simulink model "pset1_simulink"  (R2022a)
settings: Solver=VariableStepAuto  StartTime=0.0  StopTime=10.0  RelTol=1e-3
values from neighbouring files (symbols this model uses):
  a = inf    [inert2OE.m]    (also in pset1.m = state(1); pset2.m = 1 / (2 / norm(pos) - norm(vel)^2 / mu))
  e = norm(e_vec)    [inert2OE.m]    (also in pset1.m = sqrt(1 - p / a); pset2.m = sqrt(1 - p / a); pset4.m = sqrt(oe_c_mean_pert(i, 3)^2 + oe_c_mean_pert(i, 4)^2))
  i = acos(h_vec(3)/h)    [inert2OE.m]    (also in pset1.m = state(4); pset2.m = atan2(sqrt(W(1)^2 + W(2)^2), W(3)); pset5_NR.m = 1)
  mu = 3.986004418e5    (= 398600.4418)    [pset1.m]    (also in pset2.m = 398600.435436; pset3.m = 398600.435436; pset3_problem1.m = 398600.435436; pset3_problem2.m = 398600.435436)
  omega = 2*pi - omega    [inert2OE.m]    (also in pset1.m = u - nu; pset2.m = wrapTo2Pi(u - nu); pset4.m = atan2(oe_c_mean_pert(i,4), oe_c_mean_pert(i, 3)))
  RAAN = atan2(W(1), - W(2))    [pset1.m]    (also in pset2.m)
  true_anom = 0    [pset1.m]
settings Model: Creator=pauli  LastModifiedBy=pauli

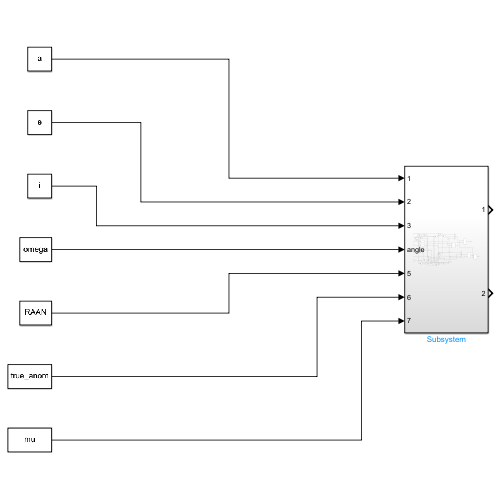
[thumbnail: Simulink's stored preview of the top-level diagram]
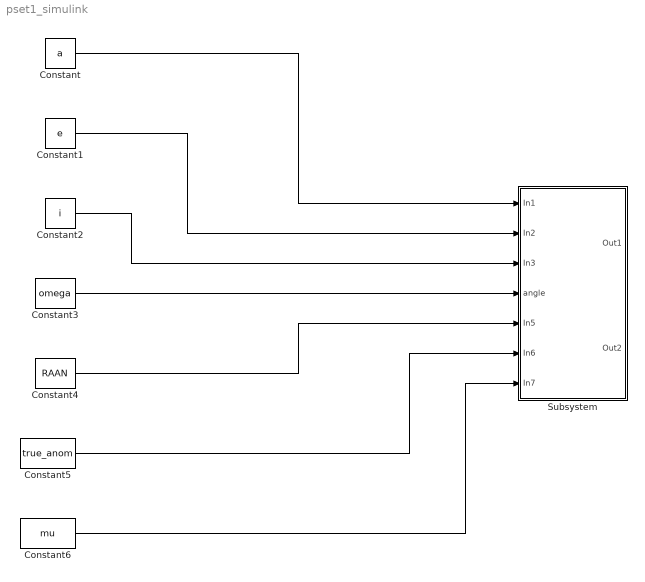
== system pset1_simulink ==
  Constant : Constant  Value=a
  Constant1 : Constant  Value=e
  Constant2 : Constant  Value=i
  Constant3 : Constant  Value=omega
  Constant4 : Constant  Value=RAAN
  Constant5 : Constant  Value=true_anom
  Constant6 : Constant  Value=mu
  Subsystem : Subsystem
  wires:
  Constant/1 -> Subsystem/1(In1)
  Constant1/1 -> Subsystem/2(In2)
  Constant2/1 -> Subsystem/3(In3)
  Constant3/1 -> Subsystem/4(angle)
  Constant4/1 -> Subsystem/5(In5)
  Constant5/1 -> Subsystem/6(In6)
  Constant6/1 -> Subsystem/7(In7)

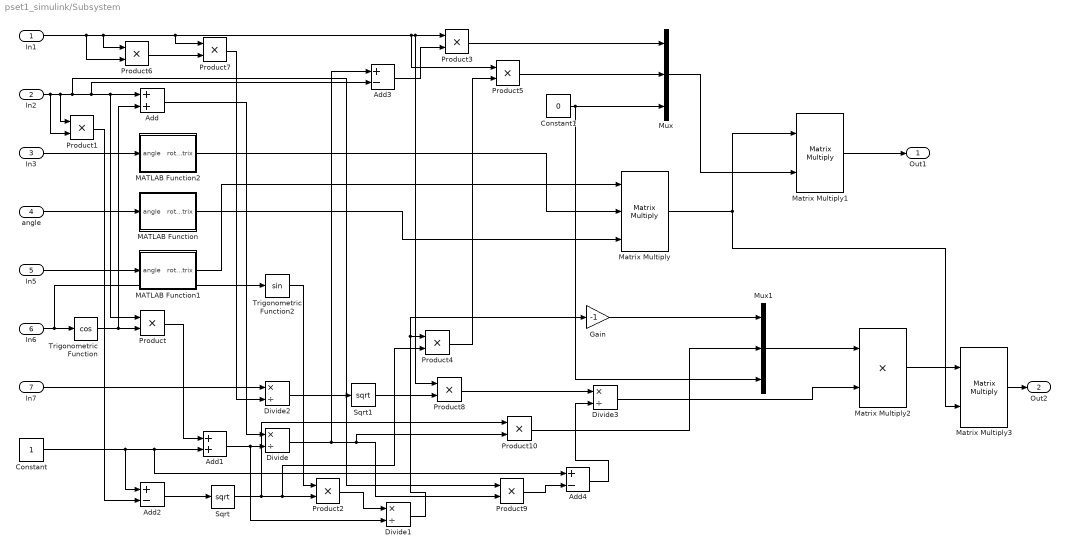
== system pset1_simulink/Subsystem ==
  In1 : Inport  Unit=km
      settings: VarSizeSig=Yes
  In2 : Inport  Port=2
  In3 : Inport  Port=3
  angle : Inport  Port=4
  In5 : Inport  Port=5
  In6 : Inport  Port=6
  In7 : Inport  Port=7
  Add : Sum
  Add1 : Sum
  Add2 : Sum  Inputs=+-
  Add3 : Sum  Inputs=+-
  Add4 : Sum  Inputs=+-
  Constant : Constant
  Constant1 : Constant  Value=0
  Divide{,1..3} (4 alike) : Product  Inputs=*/
  Gain : Gain  Gain=-1
  MATLAB Function : MATLAB Function  TreatAsAtomicUnit=on
  MATLAB Function1 : MATLAB Function  TreatAsAtomicUnit=on
  MATLAB Function2 : MATLAB Function  TreatAsAtomicUnit=on
  Matrix Multiply : Product  Inputs=3  Multiplication=Matrix(*)
  Matrix Multiply1 : Product  Multiplication=Matrix(*)
  Matrix Multiply2 : Product
  Matrix Multiply3 : Product  Multiplication=Matrix(*)
  Mux : Mux  Inputs=3
  Mux1 : Mux  Inputs=3
  Product{,1..10} (11 alike) : Product
  Sqrt : Sqrt
  Sqrt1 : Sqrt
  Trigonometric Function : Trigonometry  Operator=cos
  Trigonometric Function2 : Trigonometry
  Out1 : Outport
  Out2 : Outport  Port=2
  wires:
  In6/1 -> Trigonometric Function2/1, Trigonometric Function/1
  In2/1 -> Product1/2, Product1/1, Product9/1, Add3/2, Product/1, Add/1
  Trigonometric Function/1 -> Product/2, Add/2
  Constant/1 -> Add2/1, Add4/1, Add1/2
  Product/1 -> Add1/1
  Add1/1 -> Divide1/2, Divide/2
  Add/1 -> Divide/1
  Divide/1 -> Add3/1, Product10/2, Product9/2
  Product1/1 -> Add2/2
  Add2/1 -> Sqrt/1
  Sqrt/1 -> Product10/1, Product4/2, Product2/2
  Trigonometric Function2/1 -> Product2/1
  Product2/1 -> Divide1/1
  Divide1/1 -> Gain/1, Product4/1
  In1/1 -> Product6/2, Product6/1, Product7/1, Product8/1, Product3/1, Product5/1
  Add3/1 -> Product3/2
  Product3/1 -> Mux/1
  Product4/1 -> Product5/2
  Product5/1 -> Mux/2
  Constant1/1 -> Mux1/3, Mux/3
  angle/1 -> MATLAB Function/1(angle)
  In5/1 -> MATLAB Function1/1(angle)
  MATLAB Function1/1(rot_matrix) -> Matrix Multiply/1
  In3/1 -> MATLAB Function2/1(angle)
  MATLAB Function2/1(rot_matrix) -> Matrix Multiply/2
  MATLAB Function/1(rot_matrix) -> Matrix Multiply/3
  Matrix Multiply/1 -> Matrix Multiply3/2, Matrix Multiply1/1
  Mux/1 -> Matrix Multiply1/2
  Matrix Multiply1/1 -> Out1/1
  Product6/1 -> Product7/2
  Product7/1 -> Divide2/2
  In7/1 -> Divide2/1
  Divide2/1 -> Sqrt1/1
  Sqrt1/1 -> Product8/2
  Product9/1 -> Add4/2
  Product8/1 -> Divide3/1
  Add4/1 -> Divide3/2
  Gain/1 -> Mux1/1
  Product10/1 -> Mux1/2
  Divide3/1 -> Matrix Multiply2/2
  Mux1/1 -> Matrix Multiply2/1
  Matrix Multiply2/1 -> Matrix Multiply3/1
  Matrix Multiply3/1 -> Out2/1

== matlab function pset1_simulink/Subsystem/MATLAB Function ==
  data: angle input; rot_matrix output
function rot_matrix = rot_z(angle)
rot_matrix = eye(3);
rot_matrix(1, 1) = cos(angle);
rot_matrix(1, 2) = - sin(angle);
rot_matrix(2, 1) = sin(angle);
rot_matrix(2, 2) = cos(angle);

== matlab function pset1_simulink/Subsystem/MATLAB Function2 ==
  data: angle input; rot_matrix output
function rot_matrix = rot_x(angle)
rot_matrix = eye(3);
rot_matrix(2, 2) = cos(angle);
rot_matrix(2, 3) = - sin(angle);
rot_matrix(3, 2) = sin(angle);
rot_matrix(3, 3) = cos(angle);

== matlab function pset1_simulink/Subsystem/MATLAB Function1 ==
  data: angle input; rot_matrix output
function rot_matrix = rot_z(angle)
rot_matrix = eye(3);
rot_matrix(1, 1) = cos(angle);
rot_matrix(1, 2) = - sin(angle);
rot_matrix(2, 1) = sin(angle);
rot_matrix(2, 2) = cos(angle);
